simulink model "hysteretic_control"  (Simulink 6.1)
settings: Solver=ode23tb  StartTime=0.0  StopTime=0.04  MaxStep=1e-5  RelTol=1e-3  AbsTol=.01
libraries: powerlib x8
settings Model: LastModifiedBy=ThinkPad
settings DebuggingCC: SolverPrmCheckMsg=warning

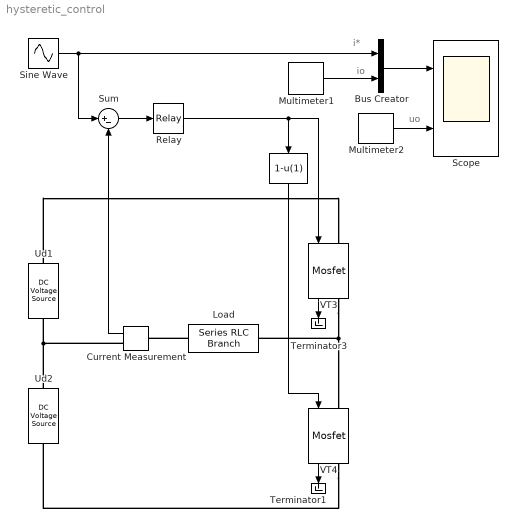
== system hysteretic_control ==
  note: uo
  note: io
  note: i*
  "  " : Fcn  Orientation=down  Expr=1-u(1)
  Bus Creator : BusCreator  DialogController=Simulink.DDGSource_Bus  Inputs=2
  Current Measurement : powerlib/Measurements/Current Measurement  Orientation=left  PhasorSimulation=off  OutputType=Complex  PSBequivalent=0
  Load : powerlib/Elements/Series RLC Branch  Orientation=left  PhysicalDomain=powersysdomain  SubClassName=unknown  LeftPortType=p1  RightPortType=p1  LConnTagsString=__new0  RConnTagsString=__new0  Resistance=1  Inductance=0.01  Capacitance=inf  Measurements=Branch voltage and current
  Multimeter1 : powerlib/Measurements/Multimeter  PhasorSimulation=off  OutputType=Complex  sel=2  L=2  Gain=1  yselected={'Ib: Load'};  PSBOutputType=1  PSBequivalent=0  AxesSetting=[0,0.1,-100,100]  Display=0  SavedBlockNames=-11
  Multimeter2 : powerlib/Measurements/Multimeter  PhasorSimulation=off  OutputType=Complex  sel=1  L=2  Gain=1  yselected={'Ub: Load'};  PSBOutputType=1  PSBequivalent=0  AxesSetting=[0,0.1,-100,100]  Display=0  SavedBlockNames=-11
  Relay : Relay  OnSwitchValue=5  OffSwitchValue=-5
  Scope : Scope  NumInputPorts=2
      settings: TimeRange=0.04  YMin=-40~-150  YMax=40~150  SampleTime=2e-4
  Sine Wave : Sin  Amplitude=20  Frequency=314  SampleTime=0
  Sum : Sum  Inputs=|+-
  Terminator1 : Terminator
      settings: Orientation=down
  Terminator3 : Terminator
      settings: Orientation=down
  Ud1 : powerlib/Electrical Sources/DC Voltage Source  Orientation=up  Amplitude=100  Measurements=None
  Ud2 : powerlib/Electrical Sources/DC Voltage Source  Orientation=up  Amplitude=100  Measurements=None
  VT3 : powerlib/Power Electronics/Mosfet  Orientation=down  Ron=0.01  Lon=1e-7  Rd=.01  IC=0  Rs=5  Cs=1e-6  Measurements=on
  VT4 : powerlib/Power Electronics/Mosfet  Orientation=down  Ron=0.01  Lon=1e-7  Rd=.01  IC=0  Rs=5  Cs=1e-6  Measurements=on
  wires:
  Relay/1 -> VT3/1, "  "/1
  VT4/1 -> Terminator1/1
  VT3/1 -> Terminator3/1
  Sine Wave/1 -> Sum/1, Bus Creator/1
  Multimeter1/1 -> Bus Creator/2
  Current Measurement/1 -> Sum/2
  Sum/1 -> Relay/1
  Bus Creator/1 -> Scope/1
  Multimeter2/1 -> Scope/2
  "  "/1 -> VT4/1
  connections:
  VT3/RConn1 -- VT4/LConn1 -- Load/LConn1
  Ud1/RConn1 -- VT3/LConn1
  Ud2/RConn1 -- Ud1/LConn1 -- Current Measurement/RConn1
  VT4/RConn1 -- Ud2/LConn1
  Load/RConn1 -- Current Measurement/LConn1
